simulink model "lon_zengwen"  (R2016a)
settings: Solver=VariableStepAuto  StartTime=0.0  StopTime=1000  RelTol=1e-3
undefined symbols (not defined in the file): Alon, Blon, Clon, Dlon
settings Model: Creator=Gray  LastModifiedBy=Gray

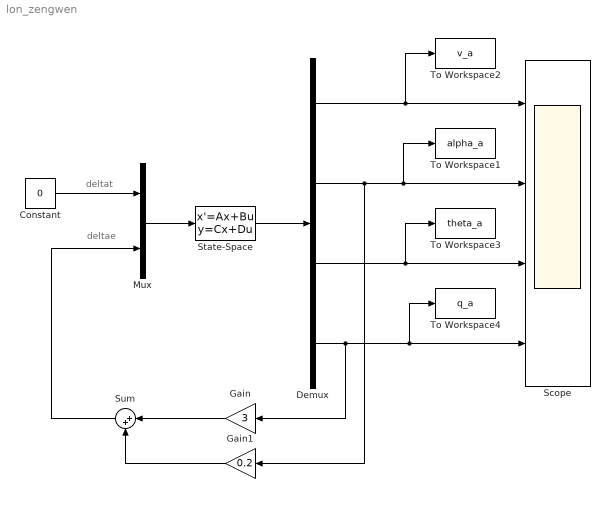
== system lon_zengwen ==
  note: deltae
  note: deltat
  Constant : Constant  Value=0
  Demux : Demux
  Gain : Gain  Gain=3
  Gain1 : Gain  Gain=0.2
  Mux : Mux  Inputs=2
  Scope : Scope  NumInputPorts=4
  State-Space : StateSpace  A=Alon  B=Blon  C=Clon  D=Dlon  X0="[0 5/57.3 0  0]'"
  Sum : Sum  Inputs=|++
  To Workspace1 : ToWorkspace  VariableName=alpha_a  SaveFormat=Timeseries  SampleTime=-1
  To Workspace2 : ToWorkspace  VariableName=v_a  SaveFormat=Timeseries  SampleTime=-1
  To Workspace3 : ToWorkspace  VariableName=theta_a  SaveFormat=Timeseries  SampleTime=-1
  To Workspace4 : ToWorkspace  VariableName=q_a  SaveFormat=Timeseries  SampleTime=-1
  wires:
  State-Space/1 -> Demux/1
  Mux/1 -> State-Space/1
  Gain1/1 -> Sum/2
  Gain/1 -> Sum/1
  Constant/1 -> Mux/1
  Sum/1 -> Mux/2
  Demux/2 -> Gain1/1, To Workspace1/1, Scope/2
  Demux/4 -> Gain/1, To Workspace4/1, Scope/4
  Demux/1 -> To Workspace2/1, Scope/1
  Demux/3 -> To Workspace3/1, Scope/3
